simulink model "test_dynamics"  (R2015b)
settings: Solver=ode3  StartTime=0.0  StopTime=10  FixedStep=0.001  RelTol=1e-12  AbsTol=0.01
values from neighbouring files (symbols this model uses):
  aeroflag = 0    [dynamics_SSM.m]
  CsInertiaModal = Aircraft.AeroelasticSSM.modeshapes'*Control_surface_inertia    [dynamics_SSM.m]
  delta_amp = 5*pi/180    (= 0.0872664625997)    [dynamics_SSM.m]
  delta_freq = 15    [dynamics_SSM.m]
  n_sines = 20    [dynamics_SSM.m]
  t_start = 0.5    [dynamics_SSM.m]
undefined symbols (not defined in the file or in its folder): Aircraft
libraries: simulink_extras x3, simulink x1
settings Model: Creator=Klaus  LastModifiedBy=rmkseywa
settings DataIOCC: SaveFormat=Array  SignalLoggingSaveFormat=ModelDataLogs
settings OptimizationCC: ExpressionDepthLimit=2147483647
settings DebuggingCC: UnderspecifiedInitializationDetection=Classic  MergeDetectMultiDrivingBlocksExec=none  SolverPrmCheckMsg=warning  MultiTaskDSMMsg=warning  MultiTaskCondExecSysMsg=none  StateNameClashWarn=warning
settings HardwareCC: ProdBitPerPointer=32  ProdLargestAtomicFloat=None  ProdIntDivRoundTo=Undefined  ProdEndianess=Unspecified  ProdWordSize=32  ProdHWDeviceType=32-bit Generic
settings GRTTargetCC: GeneratePreprocessorConditionals=Disable all
settings ConfigComp: CovModelRefEnable=Off

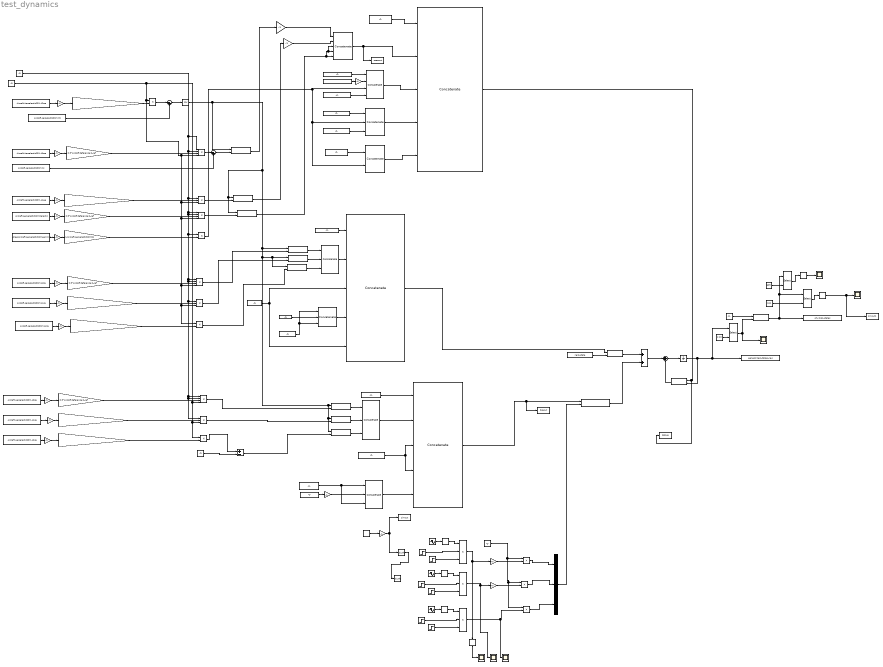
== system test_dynamics ==
  Add : Sum  Inputs=+-
  Chirp Signal : simulink/Sources/Chirp Signal  f1=0.1  T=10  f2=50
  Constant : Constant  Value=Aircraft.AeroelasticSSM.modeshapes
  Constant1 : Constant  Value=Aircraft.AeroelasticSSM.A0ee
  Constant10 : Constant  Value=-diag(Aircraft.AeroelasticSSM.gamma)
  Constant11 : Constant  Value=Aircraft.AeroelasticSSM.Eelastic  VectorParams1D=off
  Constant12 : Constant  Value=Aircraft.AeroelasticSSM.A1ee
  Constant13 : Constant  Value=[zeros(Aircraft.AeroelasticSSM.nE,Aircraft.AeroelasticSSM.nR*3)]
  Constant14 : Constant  Value=zeros(Aircraft.AeroelasticSSM.nL,Aircraft.AeroelasticSSM.nR)
  Constant15 : Constant  Value=Aircraft.AeroelasticSSM.Erigid  VectorParams1D=off
  Constant16 : Constant  Value=Aircraft.AeroelasticSSM.A0re
  Constant17 : Constant  Value=zeros(Aircraft.AeroelasticSSM.nL,Aircraft.AeroelasticSSM.nC)
  Constant18 : Constant  Value=[zeros(Aircraft.AeroelasticSSM.nL,Aircraft.AeroelasticSSM.nL*2) ]
  Constant19 : Constant  Value=Aircraft.AeroelasticSSM.A1re
  Constant2 : Constant  Value=Aircraft.AeroelasticSSM.A2ee
  Constant20 : Constant  Value=Aircraft.AeroelasticSSM.A2re
  Constant21 : Constant  Value=Aircraft.AeroelasticSSM.Econtrol  VectorParams1D=off
  Constant22 : Constant  Value=zeros(Aircraft.AeroelasticSSM.nL,Aircraft.AeroelasticSSM.nR*3)
  Constant23 : Constant  Value=Aircraft.AeroelasticSSM.A0ce
  Constant24 : Constant  Value=Aircraft.AeroelasticSSM.A1ce
  Constant25 : Constant  Value=Aircraft.AeroelasticSSM.A2ce
  Constant26 : Constant  Value=zeros(Aircraft.AeroelasticSSM.nL,Aircraft.AeroelasticSSM.nC*3)
  Constant27 : Constant  Value=[zeros(Aircraft.AeroelasticSSM.nE,Aircraft.AeroelasticSSM.nC*3)]
  Constant28 : Constant  Value=1:10
  Constant29 : Constant  Value=[zeros(Aircraft.AeroelasticSSM.nL,Aircraft.AeroelasticSSM.nL+Aircraft.AeroelasticSSM.nE*2) ]
  Constant3 : Constant  Value=Aircraft.AeroelasticSSM.Ks
  Constant30 : Constant  Value=CsInertiaModal
  Constant31 : Constant  Value=[zeros(Aircraft.AeroelasticSSM.nL,Aircraft.AeroelasticSSM.nL) ]
  Constant32 : Constant  Value=[zeros(Aircraft.AeroelasticSSM.nL,Aircraft.AeroelasticSSM.nL*2+Aircraft.AeroelasticSSM.nE*2) ]
  Constant33 : Constant  Value=[zeros(6,1); 1; zeros(4,1)]
  Constant34 : Constant  Value=609
  Constant35 : Constant  Value=611
  Constant4 : Constant  Value=Aircraft.AeroelasticSSM.Delastic
  Constant5 : Constant  Value=Aircraft.rho
  Constant6 : Constant  Value=Aircraft.V
  Constant7 : Constant  Value=[zeros(Aircraft.AeroelasticSSM.nE,Aircraft.AeroelasticSSM.nE) eye(Aircraft.AeroelasticSSM.nE,Aircraft.AeroelasticSSM.nE) zeros(Aircraft.AeroelasticSSM.nE,Aircraft.AeroelasticSSM.nL*3)]
  Constant8 : Constant  Value=zeros(Aircraft.AeroelasticSSM.nL,Aircraft.AeroelasticSSM.nE)
  Constant9 : Constant  Value=Aircraft.AeroelasticSSM.Ms
  ControlStateInputMatrix : Product  Multiplication=Matrix(*)
  Derivative : Derivative
  Derivative1 : Derivative
  From Workspace : FromWorkspace  VariableName=rigid_state  SampleTime=0  OutputAfterFinalValue=Setting to zero
  Gain{,10,15..23,25..28} (15 alike) : Gain  Gain=aeroflag
  Gain{1..2,9,11} (4 alike) : Gain  Gain=0.5*Aircraft.Reference.S_ref
  Gain12 : Gain  Gain=0.5*Aircraft.Reference.S_ref*Aircraft.AeroelasticSSM.bb
  Gain13 : Gain  Gain=0.5*Aircraft.Reference.S_ref*Aircraft.AeroelasticSSM.bb
  Gain14 : Gain  Gain=0.5*Aircraft.Reference.S_ref*Aircraft.AeroelasticSSM.bb^2
  Gain24 : Gain  Gain=5*pi/180
  Gain3 : Gain  Gain=-1
  Gain4 : Gain  Gain=-0.5*Aircraft.Reference.S_ref*Aircraft.AeroelasticSSM.bb
  Gain5 : Gain  Gain=0.5*Aircraft.Reference.S_ref*Aircraft.AeroelasticSSM.bb^2
  Gain6 : Gain  Gain=1/Aircraft.AeroelasticSSM.bb
  Gain7 : Gain  Gain=-1
  Gain8 : Gain  Gain=0.5*Aircraft.Reference.S_ref*Aircraft.AeroelasticSSM.bb^2
  Integrator : Integrator
  Matrix Concatenate{2,7..8,10..11} (5 alike) : Concatenate  NumInputs=3  Mode=Multidimensional array  ConcatenateDimension=2
  Matrix Concatenate12 : Concatenate  Mode=Multidimensional array  ConcatenateDimension=2
  Matrix Concatenate3 : Concatenate  NumInputs=5  Mode=Multidimensional array  ConcatenateDimension=2
  Matrix Concatenate4 : Concatenate  NumInputs=5  Mode=Multidimensional array
  Matrix Concatenate5 : Concatenate  NumInputs=4  Mode=Multidimensional array  ConcatenateDimension=2
  Matrix Concatenate6 : Concatenate  NumInputs=5  Mode=Multidimensional array
  Matrix Concatenate9 : Concatenate  NumInputs=5  Mode=Multidimensional array
  Mux : Mux  Inputs=3
  Product : Product  Multiplication=Matrix(*)
  Product{1,3,9..12,14..15,19} (9 alike) : Product  Multiplication=Matrix(*)  RndMeth=Zero
  Product13 : Product  Multiplication=Matrix(*)
  Product16 : Product  Inputs=3  RndMeth=Zero
  Product{2,4,17,20} (4 alike) : Product  Inputs=4  RndMeth=Zero
  Product{5,7,18,22} (4 alike) : Product  RndMeth=Zero
  Product21 : Product  Inputs=3  RndMeth=Zero
  Product23 : Product  Multiplication=Matrix(*)
  Product24 : Product  Inputs=3
  Product25 : Product  Inputs=3
  Product26 : Product  Inputs=3
  Product27 : Product
  Product28 : Product
  Product29 : Product
  Product6 : Product  Inputs=3  RndMeth=Zero
  Product8 : Product  Inputs=/  Multiplication=Matrix(*)
  Radians to Degrees : simulink_extras/Transformations/Radians to Degrees
  Radians to Degrees1 : simulink_extras/Transformations/Radians to Degrees
  Radians to Degrees2 : simulink_extras/Transformations/Radians to Degrees
  Scope{,1..5} (6 alike) : Scope
  Selector : Selector  InputPortWidth=56  IndexOptions=Index vector (port)  Indices=[1 3]  OutputSizes=1
  Selector1 : Selector  InputPortWidth=612  IndexOptions=Index vector (port)  Indices=[1 3]  OutputSizes=1
  Selector2 : Selector  InputPortWidth=612  IndexOptions=Index vector (port)  Indices=[1 3]  OutputSizes=1
  Sine Wave : Sin  Amplitude=delta_amp  Frequency=delta_freq*2*pi  SampleTime=0
  Sine Wave1 : Sin  Amplitude=delta_freq*2*pi*delta_amp  Frequency=delta_freq*2*pi  Phase=pi/2  SampleTime=0
  Sine Wave2 : Sin  Amplitude=delta_freq*2*pi*delta_amp*delta_freq*2*pi  Frequency=delta_freq*2*pi  Phase=pi  SampleTime=0
  Step : Step  Time=t_start  SampleTime=0
  Step1 : Step  Time=t_start+n_sines/delta_freq  Before=1  After=0  SampleTime=0
  Step2 : Step  Time=t_start  SampleTime=0
  Step3 : Step  Time=t_start+n_sines/delta_freq  Before=1  After=0  SampleTime=0
  Step4 : Step  Time=t_start  SampleTime=0
  Step5 : Step  Time=t_start+n_sines/delta_freq  Before=1  After=0  SampleTime=0
  Sum : Sum  Inputs=|++
  Sum1 : Sum  Inputs=|-+
  Sum2 : Sum  Inputs=|-+
  Sum3 : Sum
  To Workspace : ToWorkspace  VariableName=generalized_states_new  SaveFormat=Timeseries  SampleTime=-1
  To Workspace1 : ToWorkspace  VariableName=physical_states  SaveFormat=Timeseries  SampleTime=-1
  To Workspace2 : ToWorkspace  VariableName=bceout  SaveFormat=Timeseries  SampleTime=-1
  To Workspace3 : ToWorkspace  VariableName=aseeout  SaveFormat=Timeseries  SampleTime=-1
  To Workspace4 : ToWorkspace  VariableName=debug  SaveFormat=Timeseries  SampleTime=-1
  To Workspace5 : ToWorkspace  VariableName=simout  SaveFormat=Timeseries  SampleTime=-1
  To Workspace6 : ToWorkspace  VariableName=simout1  SaveFormat=Timeseries  SampleTime=-1
  Transport Delay : TransportDelay  DelayTime=t_start
  Transport Delay1 : TransportDelay  DelayTime=t_start
  Transport Delay2 : TransportDelay  DelayTime=t_start
  wires:
  Sum/1 -> Integrator/1
  Product13/1 -> Sum/2
  Constant16/1 -> Gain18/1
  Constant19/1 -> Gain19/1
  Gain11/1 -> Product17/3
  Gain12/1 -> Product16/2
  Constant20/1 -> Gain20/1
  Gain8/1 -> Product18/2
  Constant13/1 -> Matrix Concatenate6/1
  Product10/1 -> Matrix Concatenate7/1
  Product11/1 -> Matrix Concatenate7/2
  Matrix Concatenate7/1 -> Matrix Concatenate6/2
  Constant15/1 -> Matrix Concatenate8/2
  Matrix Concatenate8/1 -> Matrix Concatenate6/4
  Product12/1 -> Matrix Concatenate7/3
  Constant14/1 -> Matrix Concatenate8/1, Matrix Concatenate8/3
  Constant22/1 -> Matrix Concatenate6/5, Matrix Concatenate6/3
  Product17/1 -> Product10/2  "V*V*0.5*S_ref*A0re"
  Product16/1 -> Product11/2
  Product18/1 -> Product12/2
  Product7/1 -> Sum1/1
  Sum1/1 -> Product8/1
  Constant9/1 -> Sum1/2
  Gain5/1 -> Product7/2
  Matrix Concatenate6/1 -> Product/1
  From Workspace/1 -> Product/2
  Constant3/1 -> Sum2/2
  Product4/1 -> Sum2/1
  Sum2/1 -> Product1/2  "Kaee"
  Constant12/1 -> Gain10/1
  Constant4/1 -> Gain15/1
  Product2/1 -> Product9/2
  Product6/1 -> Product3/2  "Caee"
  Constant10/1 -> Gain16/1
  Gain6/1 -> Product5/2
  Product8/1 -> Product1/1, Product9/1, Product3/1, Product12/1, Product11/1, Product19/1, Product15/1, Product14/1, Product10/1
  Product5/1 -> Matrix Concatenate5/3, Matrix Concatenate12/2, Matrix Concatenate2/2
  Gain3/1 -> Matrix Concatenate3/1
  Gain7/1 -> Matrix Concatenate3/2
  Constant7/1 -> Matrix Concatenate4/1
  Constant11/1 -> Gain26/1
  Matrix Concatenate3/1 -> To Workspace3/1, Matrix Concatenate4/2
  Constant8/1 -> Matrix Concatenate5/1
  Constant18/1 -> Matrix Concatenate5/4
  Constant29/1 -> Matrix Concatenate2/1
  Constant31/1 -> Matrix Concatenate2/3
  Constant32/1 -> Matrix Concatenate12/1
  Product9/1 -> Matrix Concatenate3/3, Matrix Concatenate3/4, Matrix Concatenate3/5
  Product3/1 -> Gain7/1
  Product1/1 -> Gain3/1
  Constant1/1 -> Gain/1
  ControlStateInputMatrix/1 -> Sum3/2
  Matrix Concatenate9/1 -> To Workspace2/1, ControlStateInputMatrix/1
  Sum3/1 -> Sum/1
  Constant27/1 -> Matrix Concatenate9/1
  Constant17/1 -> Matrix Concatenate11/3, Matrix Concatenate11/1
  Constant21/1 -> Gain25/1
  Constant6/1 -> Product4/1, Product4/2, Product20/1, Product20/2, Product21/1, Product16/1, Product17/2, Product17/1, Product5/1, Product2/2, Product2/1, Product6/1
  Constant5/1 -> Product20/4, Product22/1, Product21/3, Product4/4, Product18/1, Product16/3, Product17/4, Product2/4, Product6/3, Product7/1
  Constant23/1 -> Gain21/1
  Constant24/1 -> Gain22/1
  Constant25/1 -> Gain23/1
  Matrix Concatenate10/1 -> Matrix Concatenate9/2
  Matrix Concatenate11/1 -> Matrix Concatenate9/5
  Product14/1 -> Matrix Concatenate10/1
  Product15/1 -> Matrix Concatenate10/2
  Product19/1 -> Matrix Concatenate10/3
  Constant26/1 -> Matrix Concatenate9/4, Matrix Concatenate9/3
  Gain9/1 -> Product20/3
  Gain13/1 -> Product21/2
  Gain14/1 -> Product22/2
  Product20/1 -> Product14/2
  Product21/1 -> Product15/2
  Product22/1 -> Add/1
  Constant/1 -> Product23/1
  Selector/1 -> Product23/2, Scope1/1
  Integrator/1 -> Product13/2, To Workspace/1, Selector/1
  Constant28/1 -> Selector/2
  Step/1 -> Product24/2
  Step1/1 -> Product24/3
  Sine Wave/1 -> Transport Delay/1
  Transport Delay/1 -> Product24/1
  Step2/1 -> Product25/2
  Step3/1 -> Product25/3
  Sine Wave1/1 -> Transport Delay1/1
  Transport Delay1/1 -> Product25/1
  Product25/1 -> Gain28/1, Scope3/1
  Step4/1 -> Product26/2
  Step5/1 -> Product26/3
  Sine Wave2/1 -> Transport Delay2/1
  Transport Delay2/1 -> Product26/1
  Constant33/1 -> Product29/1, Product28/1, Product27/1
  Product29/1 -> Mux/3
  Mux/1 -> ControlStateInputMatrix/2
  Constant30/1 -> Add/2
  Add/1 -> Product19/2
  Constant34/1 -> Selector1/2
  Selector1/1 -> Radians to Degrees/1
  Matrix Concatenate4/1 -> To Workspace4/1, Product13/1
  Matrix Concatenate5/1 -> Matrix Concatenate4/3
  Matrix Concatenate2/1 -> Matrix Concatenate4/4
  Matrix Concatenate12/1 -> Matrix Concatenate4/5
  Product24/1 -> Gain27/1, Radians to Degrees1/1
  Product27/1 -> Mux/1
  Gain1/1 -> Product4/3
  Constant2/1 -> Gain17/1
  Gain4/1 -> Product6/2
  Gain2/1 -> Product2/3
  Product28/1 -> Mux/2
  Product23/1 -> Selector1/1, Selector2/1, To Workspace1/1
  Constant35/1 -> Selector2/2
  Selector2/1 -> Radians to Degrees2/1
  Radians to Degrees/1 -> Scope2/1
  Gain/1 -> Gain1/1
  Gain10/1 -> Gain4/1
  Gain15/1 -> Gain2/1
  Gain16/1 -> Gain6/1
  Gain17/1 -> Gain5/1
  Radians to Degrees1/1 -> Scope/1
  Radians to Degrees2/1 -> To Workspace6/1, Scope4/1
  Gain18/1 -> Gain11/1
  Gain19/1 -> Gain12/1
  Gain20/1 -> Gain8/1
  Gain21/1 -> Gain9/1
  Gain22/1 -> Gain13/1
  Gain23/1 -> Gain14/1
  Chirp Signal/1 -> Gain24/1
  Gain24/1 -> To Workspace5/1, Derivative/1
  Derivative/1 -> Derivative1/1
  Product26/1 -> Scope5/1, Product29/2
  Gain25/1 -> Matrix Concatenate11/2
  Gain26/1 -> Matrix Concatenate5/2
  Product/1 -> Sum3/1
  Gain27/1 -> Product27/2
  Gain28/1 -> Product28/2
